simulink model "untitled"  (R2024a)
settings: Solver=VariableStepAuto  StartTime=0.0  StopTime=10.0  RelTol=1e-3
undefined symbols (not defined in the file): x
settings Model: Creator=Hulumulu  LastModifiedBy=Hulumulu

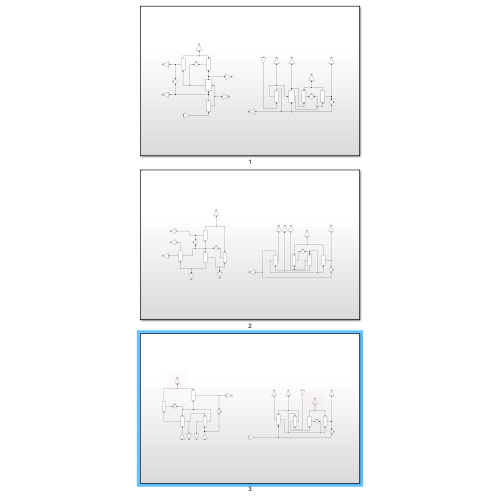
[thumbnail: Simulink's stored preview of the top-level diagram]
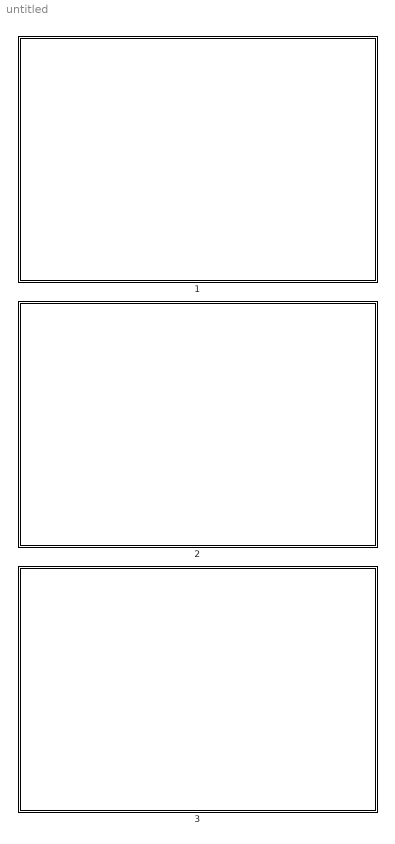
== system untitled ==
  1 : Subsystem
  2 : Subsystem
  3 : Subsystem

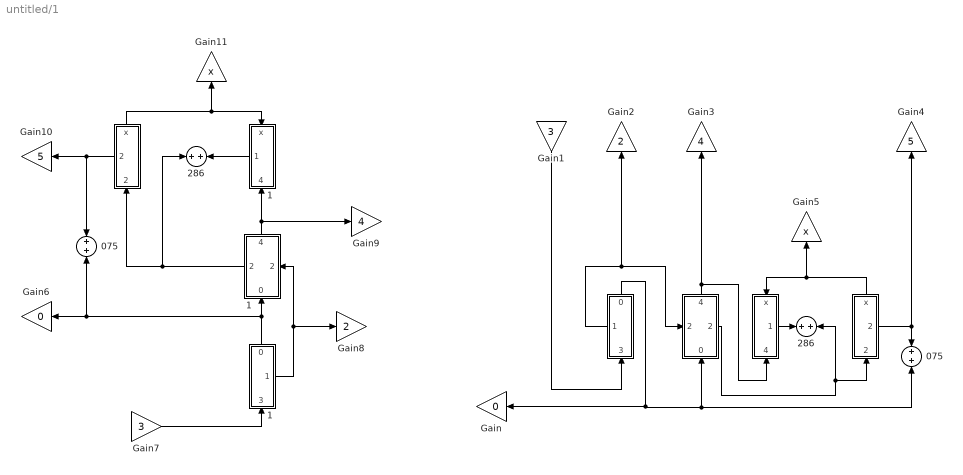
== system untitled/1 ==
  " " : Subsystem
      settings: PortSchema="{\"entries\":[{\"content\":{\"sides\":[{\"content\":{},\"type\":\"ConnectorPlacement.EquallySpacedRectSide\",\"uuid\":\"fb5bb639-39a6-4afc-972d-2ab36dd157e3\"},{\"content\":{\"connectorIds\":[\"Out1\"],\"side\":\"RIGHT\"},\"type\":\"ConnectorPlacement.EquallySpacedRectSide\",\"uuid\":\"d36a19b9-286f-415f-8446-30942908938a\"},{\"content\":{\"connectorIds\":[\"Out2\"],\"side\":\"TOP\"},\"type\":\"ConnectorPlacement.EquallySpacedRectSide\",\"uuid\":\"8c87528f-8b9e-42ba-b050-7318306b7d2b\"},{\"content\":{\"connectorIds\":[\"In1\"],\"side\":\"BOTTOM\"},\"type\":\"ConnectorPlacement.EquallySpacedRectSide\",\"uuid\":\"c4959390-5d76-48db-85f4-dc53d81287e7\"}]},\"type\":\"ConnectorPlacement.EquallySpacedConnector\",\"uuid\":\"3c6f580a-50c2-42c3-8feb-567ef8b292c6\"}],\"packageUris\":[\"http://schema.mathworks.com/mf0/Connector/R2020b\"],\"version\":\"1.0\"}"
  "  " : Subsystem
      settings: PortSchema="{\"entries\":[{\"content\":{\"sides\":[{\"content\":{\"connectorIds\":[\"Out2\"]},\"type\":\"ConnectorPlacement.EquallySpacedRectSide\",\"uuid\":\"fb5bb639-39a6-4afc-972d-2ab36dd157e3\"},{\"content\":{\"connectorIds\":[\"In2\"],\"side\":\"RIGHT\"},\"type\":\"ConnectorPlacement.EquallySpacedRectSide\",\"uuid\":\"d36a19b9-286f-415f-8446-30942908938a\"},{\"content\":{\"connectorIds\":[\"Out1\"],\"side\":\"TOP\"},\"type\":\"ConnectorPlacement.EquallySpacedRectSide\",\"uuid\":\"8c87528f-8b9e-42ba-b050-7318306b7d2b\"},{\"content\":{\"connectorIds\":[\"In1\"],\"side\":\"BOTTOM\"},\"type\":\"ConnectorPlacement.EquallySpacedRectSide\",\"uuid\":\"c4959390-5d76-48db-85f4-dc53d81287e7\"}]},\"type\":\"ConnectorPlacement.EquallySpacedConnector\",\"uuid\":\"3c6f580a-50c2-42c3-8feb-567ef8b292c6\"}],\"packageUris\":[\"http://schema.mathworks.com/mf0/Connector/R2020b\"],\"version\":\"1.0\"}"
  "   " : Subsystem
      settings: PortSchema="{\"entries\":[{\"content\":{\"sides\":[{\"content\":{\"connectorIds\":[\"Out1\"]},\"type\":\"ConnectorPlacement.EquallySpacedRectSide\",\"uuid\":\"fb5bb639-39a6-4afc-972d-2ab36dd157e3\"},{\"content\":{\"side\":\"RIGHT\"},\"type\":\"ConnectorPlacement.EquallySpacedRectSide\",\"uuid\":\"d36a19b9-286f-415f-8446-30942908938a\"},{\"content\":{\"connectorIds\":[\"In1\"],\"side\":\"TOP\"},\"type\":\"ConnectorPlacement.EquallySpacedRectSide\",\"uuid\":\"8c87528f-8b9e-42ba-b050-7318306b7d2b\"},{\"content\":{\"connectorIds\":[\"In2\"],\"side\":\"BOTTOM\"},\"type\":\"ConnectorPlacement.EquallySpacedRectSide\",\"uuid\":\"c4959390-5d76-48db-85f4-dc53d81287e7\"}]},\"type\":\"ConnectorPlacement.EquallySpacedConnector\",\"uuid\":\"3c6f580a-50c2-42c3-8feb-567ef8b292c6\"}],\"packageUris\":[\"http://schema.mathworks.com/mf0/Connector/R2020b\"],\"version\":\"1.0\"}"
  "    " : Subsystem
      settings: PortSchema="{\"entries\":[{\"content\":{\"sides\":[{\"content\":{\"connectorIds\":[\"Out2\"]},\"type\":\"ConnectorPlacement.EquallySpacedRectSide\",\"uuid\":\"fb5bb639-39a6-4afc-972d-2ab36dd157e3\"},{\"content\":{\"side\":\"RIGHT\"},\"type\":\"ConnectorPlacement.EquallySpacedRectSide\",\"uuid\":\"d36a19b9-286f-415f-8446-30942908938a\"},{\"content\":{\"connectorIds\":[\"Out1\"],\"side\":\"TOP\"},\"type\":\"ConnectorPlacement.EquallySpacedRectSide\",\"uuid\":\"8c87528f-8b9e-42ba-b050-7318306b7d2b\"},{\"content\":{\"connectorIds\":[\"In1\"],\"side\":\"BOTTOM\"},\"type\":\"ConnectorPlacement.EquallySpacedRectSide\",\"uuid\":\"c4959390-5d76-48db-85f4-dc53d81287e7\"}]},\"type\":\"ConnectorPlacement.EquallySpacedConnector\",\"uuid\":\"3c6f580a-50c2-42c3-8feb-567ef8b292c6\"}],\"packageUris\":[\"http://schema.mathworks.com/mf0/Connector/R2020b\"],\"version\":\"1.0\"}"
  "     " : Subsystem
      settings: PortSchema="{\"entries\":[{\"content\":{\"sides\":[{\"content\":{\"connectorIds\":[\"Out2\"]},\"type\":\"ConnectorPlacement.EquallySpacedRectSide\",\"uuid\":\"fb5bb639-39a6-4afc-972d-2ab36dd157e3\"},{\"content\":{\"side\":\"RIGHT\"},\"type\":\"ConnectorPlacement.EquallySpacedRectSide\",\"uuid\":\"d36a19b9-286f-415f-8446-30942908938a\"},{\"content\":{\"connectorIds\":[\"Out1\"],\"side\":\"TOP\"},\"type\":\"ConnectorPlacement.EquallySpacedRectSide\",\"uuid\":\"8c87528f-8b9e-42ba-b050-7318306b7d2b\"},{\"content\":{\"connectorIds\":[\"In1\"],\"side\":\"BOTTOM\"},\"type\":\"ConnectorPlacement.EquallySpacedRectSide\",\"uuid\":\"c4959390-5d76-48db-85f4-dc53d81287e7\"}]},\"type\":\"ConnectorPlacement.EquallySpacedConnector\",\"uuid\":\"3c6f580a-50c2-42c3-8feb-567ef8b292c6\"}],\"packageUris\":[\"http://schema.mathworks.com/mf0/Connector/R2020b\"],\"version\":\"1.0\"}"
  "   1" : Subsystem
      settings: PortSchema="{\"entries\":[{\"content\":{\"sides\":[{\"content\":{\"connectorIds\":[\"Out1\"]},\"type\":\"ConnectorPlacement.EquallySpacedRectSide\",\"uuid\":\"fb5bb639-39a6-4afc-972d-2ab36dd157e3\"},{\"content\":{\"side\":\"RIGHT\"},\"type\":\"ConnectorPlacement.EquallySpacedRectSide\",\"uuid\":\"d36a19b9-286f-415f-8446-30942908938a\"},{\"content\":{\"connectorIds\":[\"In1\"],\"side\":\"TOP\"},\"type\":\"ConnectorPlacement.EquallySpacedRectSide\",\"uuid\":\"8c87528f-8b9e-42ba-b050-7318306b7d2b\"},{\"content\":{\"connectorIds\":[\"In2\"],\"side\":\"BOTTOM\"},\"type\":\"ConnectorPlacement.EquallySpacedRectSide\",\"uuid\":\"c4959390-5d76-48db-85f4-dc53d81287e7\"}]},\"type\":\"ConnectorPlacement.EquallySpacedConnector\",\"uuid\":\"3c6f580a-50c2-42c3-8feb-567ef8b292c6\"}],\"packageUris\":[\"http://schema.mathworks.com/mf0/Connector/R2020b\"],\"version\":\"1.0\"}"
  "  1" : Subsystem
      settings: PortSchema="{\"entries\":[{\"content\":{\"sides\":[{\"content\":{\"connectorIds\":[\"Out2\"]},\"type\":\"ConnectorPlacement.EquallySpacedRectSide\",\"uuid\":\"fb5bb639-39a6-4afc-972d-2ab36dd157e3\"},{\"content\":{\"connectorIds\":[\"In2\"],\"side\":\"RIGHT\"},\"type\":\"ConnectorPlacement.EquallySpacedRectSide\",\"uuid\":\"d36a19b9-286f-415f-8446-30942908938a\"},{\"content\":{\"connectorIds\":[\"Out1\"],\"side\":\"TOP\"},\"type\":\"ConnectorPlacement.EquallySpacedRectSide\",\"uuid\":\"8c87528f-8b9e-42ba-b050-7318306b7d2b\"},{\"content\":{\"connectorIds\":[\"In1\"],\"side\":\"BOTTOM\"},\"type\":\"ConnectorPlacement.EquallySpacedRectSide\",\"uuid\":\"c4959390-5d76-48db-85f4-dc53d81287e7\"}]},\"type\":\"ConnectorPlacement.EquallySpacedConnector\",\"uuid\":\"3c6f580a-50c2-42c3-8feb-567ef8b292c6\"}],\"packageUris\":[\"http://schema.mathworks.com/mf0/Connector/R2020b\"],\"version\":\"1.0\"}"
  " 1" : Subsystem
      settings: PortSchema="{\"entries\":[{\"content\":{\"sides\":[{\"content\":{},\"type\":\"ConnectorPlacement.EquallySpacedRectSide\",\"uuid\":\"fb5bb639-39a6-4afc-972d-2ab36dd157e3\"},{\"content\":{\"connectorIds\":[\"Out1\"],\"side\":\"RIGHT\"},\"type\":\"ConnectorPlacement.EquallySpacedRectSide\",\"uuid\":\"d36a19b9-286f-415f-8446-30942908938a\"},{\"content\":{\"connectorIds\":[\"Out2\"],\"side\":\"TOP\"},\"type\":\"ConnectorPlacement.EquallySpacedRectSide\",\"uuid\":\"8c87528f-8b9e-42ba-b050-7318306b7d2b\"},{\"content\":{\"connectorIds\":[\"In1\"],\"side\":\"BOTTOM\"},\"type\":\"ConnectorPlacement.EquallySpacedRectSide\",\"uuid\":\"c4959390-5d76-48db-85f4-dc53d81287e7\"}]},\"type\":\"ConnectorPlacement.EquallySpacedConnector\",\"uuid\":\"3c6f580a-50c2-42c3-8feb-567ef8b292c6\"}],\"packageUris\":[\"http://schema.mathworks.com/mf0/Connector/R2020b\"],\"version\":\"1.0\"}"
  075 : Sum  Inputs=+|+
  "075 " : Sum  Inputs=+|+
  286 : Sum  Inputs=+|+
  "286 " : Sum  Inputs=+|+
  Gain : Gain  Gain=0
  Gain1 : Gain  Gain=3
  Gain10 : Gain  Gain=5
  Gain11 : Gain  Gain=x
  Gain2 : Gain  Gain=2
  Gain3 : Gain  Gain=4
  Gain4 : Gain  Gain=5
  Gain5 : Gain  Gain=x
  Gain6 : Gain  Gain=0
  Gain7 : Gain  Gain=3
  Gain8 : Gain  Gain=2
  Gain9 : Gain  Gain=4
  wires:
  " "/1(2) -> "  "/2("2 "), Gain2/1
  "  "/2(2) -> "    "/1(2), 286/2
  "  "/1(4) -> "   "/2(4), Gain3/1
  "    "/1(x) -> Gain5/1, "   "/1(x)
  Gain1/1 -> " "/1(3)
  "   "/1(6) -> 286/1
  "    "/2(5) -> Gain4/1, 075/1
  " "/2(0) -> "  "/1(0), 075/2, Gain/1
  Gain7/1 -> " 1"/1(3)
  "     "/2(5) -> "075 "/1, Gain10/1
  "   1"/1(6) -> "286 "/2
  "  1"/1(4) -> Gain9/1, "   1"/2(4)
  "     "/1(x) -> Gain11/1, "   1"/1(x)
  " 1"/1(2) -> "  1"/2("2 "), Gain8/1
  " 1"/2(0) -> "075 "/2, Gain6/1, "  1"/1(0)
  "  1"/2(2) -> "286 "/1, "     "/1(2)

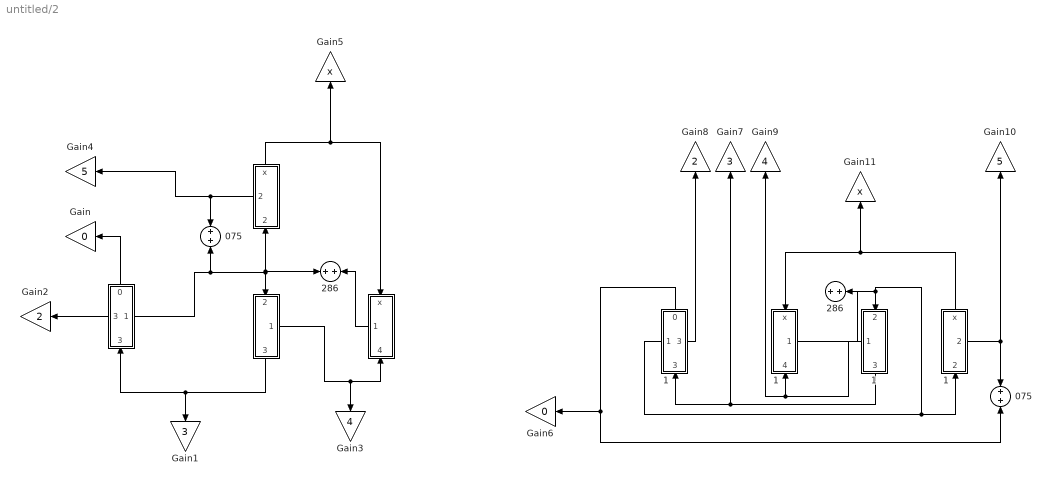
== system untitled/2 ==
  " " : Subsystem
      settings: PortSchema="{\"entries\":[{\"content\":{\"sides\":[{\"content\":{\"connectorIds\":[\"Out3\"]},\"type\":\"ConnectorPlacement.EquallySpacedRectSide\",\"uuid\":\"fb5bb639-39a6-4afc-972d-2ab36dd157e3\"},{\"content\":{\"connectorIds\":[\"Out1\"],\"side\":\"RIGHT\"},\"type\":\"ConnectorPlacement.EquallySpacedRectSide\",\"uuid\":\"d36a19b9-286f-415f-8446-30942908938a\"},{\"content\":{\"connectorIds\":[\"Out2\"],\"side\":\"TOP\"},\"type\":\"ConnectorPlacement.EquallySpacedRectSide\",\"uuid\":\"8c87528f-8b9e-42ba-b050-7318306b7d2b\"},{\"content\":{\"connectorIds\":[\"In1\"],\"side\":\"BOTTOM\"},\"type\":\"ConnectorPlacement.EquallySpacedRectSide\",\"uuid\":\"c4959390-5d76-48db-85f4-dc53d81287e7\"}]},\"type\":\"ConnectorPlacement.EquallySpacedConnector\",\"uuid\":\"3c6f580a-50c2-42c3-8feb-567ef8b292c6\"}],\"packageUris\":[\"http://schema.mathworks.com/mf0/Connector/R2020b\"],\"version\":\"1.0\"}"
  "   " : Subsystem
      settings: PortSchema="{\"entries\":[{\"content\":{\"sides\":[{\"content\":{\"connectorIds\":[\"Out1\"]},\"type\":\"ConnectorPlacement.EquallySpacedRectSide\",\"uuid\":\"fb5bb639-39a6-4afc-972d-2ab36dd157e3\"},{\"content\":{\"side\":\"RIGHT\"},\"type\":\"ConnectorPlacement.EquallySpacedRectSide\",\"uuid\":\"d36a19b9-286f-415f-8446-30942908938a\"},{\"content\":{\"connectorIds\":[\"In1\"],\"side\":\"TOP\"},\"type\":\"ConnectorPlacement.EquallySpacedRectSide\",\"uuid\":\"8c87528f-8b9e-42ba-b050-7318306b7d2b\"},{\"content\":{\"connectorIds\":[\"In2\"],\"side\":\"BOTTOM\"},\"type\":\"ConnectorPlacement.EquallySpacedRectSide\",\"uuid\":\"c4959390-5d76-48db-85f4-dc53d81287e7\"}]},\"type\":\"ConnectorPlacement.EquallySpacedConnector\",\"uuid\":\"3c6f580a-50c2-42c3-8feb-567ef8b292c6\"}],\"packageUris\":[\"http://schema.mathworks.com/mf0/Connector/R2020b\"],\"version\":\"1.0\"}"
  "    " : Subsystem
      settings: PortSchema="{\"entries\":[{\"content\":{\"sides\":[{\"content\":{\"connectorIds\":[\"Out2\"]},\"type\":\"ConnectorPlacement.EquallySpacedRectSide\",\"uuid\":\"fb5bb639-39a6-4afc-972d-2ab36dd157e3\"},{\"content\":{\"side\":\"RIGHT\"},\"type\":\"ConnectorPlacement.EquallySpacedRectSide\",\"uuid\":\"d36a19b9-286f-415f-8446-30942908938a\"},{\"content\":{\"connectorIds\":[\"Out1\"],\"side\":\"TOP\"},\"type\":\"ConnectorPlacement.EquallySpacedRectSide\",\"uuid\":\"8c87528f-8b9e-42ba-b050-7318306b7d2b\"},{\"content\":{\"connectorIds\":[\"In1\"],\"side\":\"BOTTOM\"},\"type\":\"ConnectorPlacement.EquallySpacedRectSide\",\"uuid\":\"c4959390-5d76-48db-85f4-dc53d81287e7\"}]},\"type\":\"ConnectorPlacement.EquallySpacedConnector\",\"uuid\":\"3c6f580a-50c2-42c3-8feb-567ef8b292c6\"}],\"packageUris\":[\"http://schema.mathworks.com/mf0/Connector/R2020b\"],\"version\":\"1.0\"}"
  "     " : Subsystem
      settings: PortSchema="{\"entries\":[{\"content\":{\"sides\":[{\"content\":{},\"type\":\"ConnectorPlacement.EquallySpacedRectSide\",\"uuid\":\"fb5bb639-39a6-4afc-972d-2ab36dd157e3\"},{\"content\":{\"connectorIds\":[\"Out1\"],\"side\":\"RIGHT\"},\"type\":\"ConnectorPlacement.EquallySpacedRectSide\",\"uuid\":\"d36a19b9-286f-415f-8446-30942908938a\"},{\"content\":{\"connectorIds\":[\"In1\"],\"side\":\"TOP\"},\"type\":\"ConnectorPlacement.EquallySpacedRectSide\",\"uuid\":\"8c87528f-8b9e-42ba-b050-7318306b7d2b\"},{\"content\":{\"connectorIds\":[\"Out2\"],\"side\":\"BOTTOM\"},\"type\":\"ConnectorPlacement.EquallySpacedRectSide\",\"uuid\":\"c4959390-5d76-48db-85f4-dc53d81287e7\"}]},\"type\":\"ConnectorPlacement.EquallySpacedConnector\",\"uuid\":\"3c6f580a-50c2-42c3-8feb-567ef8b292c6\"}],\"packageUris\":[\"http://schema.mathworks.com/mf0/Connector/R2020b\"],\"version\":\"1.0\"}"
  "     1" : Subsystem
      settings: PortSchema="{\"entries\":[{\"content\":{\"sides\":[{\"content\":{},\"type\":\"ConnectorPlacement.EquallySpacedRectSide\",\"uuid\":\"fb5bb639-39a6-4afc-972d-2ab36dd157e3\"},{\"content\":{\"connectorIds\":[\"Out1\"],\"side\":\"RIGHT\"},\"type\":\"ConnectorPlacement.EquallySpacedRectSide\",\"uuid\":\"d36a19b9-286f-415f-8446-30942908938a\"},{\"content\":{\"connectorIds\":[\"In1\"],\"side\":\"TOP\"},\"type\":\"ConnectorPlacement.EquallySpacedRectSide\",\"uuid\":\"8c87528f-8b9e-42ba-b050-7318306b7d2b\"},{\"content\":{\"connectorIds\":[\"Out2\"],\"side\":\"BOTTOM\"},\"type\":\"ConnectorPlacement.EquallySpacedRectSide\",\"uuid\":\"c4959390-5d76-48db-85f4-dc53d81287e7\"}]},\"type\":\"ConnectorPlacement.EquallySpacedConnector\",\"uuid\":\"3c6f580a-50c2-42c3-8feb-567ef8b292c6\"}],\"packageUris\":[\"http://schema.mathworks.com/mf0/Connector/R2020b\"],\"version\":\"1.0\"}"
  "    1" : Subsystem
      settings: PortSchema="{\"entries\":[{\"content\":{\"sides\":[{\"content\":{\"connectorIds\":[\"Out2\"]},\"type\":\"ConnectorPlacement.EquallySpacedRectSide\",\"uuid\":\"fb5bb639-39a6-4afc-972d-2ab36dd157e3\"},{\"content\":{\"side\":\"RIGHT\"},\"type\":\"ConnectorPlacement.EquallySpacedRectSide\",\"uuid\":\"d36a19b9-286f-415f-8446-30942908938a\"},{\"content\":{\"connectorIds\":[\"Out1\"],\"side\":\"TOP\"},\"type\":\"ConnectorPlacement.EquallySpacedRectSide\",\"uuid\":\"8c87528f-8b9e-42ba-b050-7318306b7d2b\"},{\"content\":{\"connectorIds\":[\"In1\"],\"side\":\"BOTTOM\"},\"type\":\"ConnectorPlacement.EquallySpacedRectSide\",\"uuid\":\"c4959390-5d76-48db-85f4-dc53d81287e7\"}]},\"type\":\"ConnectorPlacement.EquallySpacedConnector\",\"uuid\":\"3c6f580a-50c2-42c3-8feb-567ef8b292c6\"}],\"packageUris\":[\"http://schema.mathworks.com/mf0/Connector/R2020b\"],\"version\":\"1.0\"}"
  "   1" : Subsystem
      settings: PortSchema="{\"entries\":[{\"content\":{\"sides\":[{\"content\":{\"connectorIds\":[\"Out1\"]},\"type\":\"ConnectorPlacement.EquallySpacedRectSide\",\"uuid\":\"fb5bb639-39a6-4afc-972d-2ab36dd157e3\"},{\"content\":{\"side\":\"RIGHT\"},\"type\":\"ConnectorPlacement.EquallySpacedRectSide\",\"uuid\":\"d36a19b9-286f-415f-8446-30942908938a\"},{\"content\":{\"connectorIds\":[\"In1\"],\"side\":\"TOP\"},\"type\":\"ConnectorPlacement.EquallySpacedRectSide\",\"uuid\":\"8c87528f-8b9e-42ba-b050-7318306b7d2b\"},{\"content\":{\"connectorIds\":[\"In2\"],\"side\":\"BOTTOM\"},\"type\":\"ConnectorPlacement.EquallySpacedRectSide\",\"uuid\":\"c4959390-5d76-48db-85f4-dc53d81287e7\"}]},\"type\":\"ConnectorPlacement.EquallySpacedConnector\",\"uuid\":\"3c6f580a-50c2-42c3-8feb-567ef8b292c6\"}],\"packageUris\":[\"http://schema.mathworks.com/mf0/Connector/R2020b\"],\"version\":\"1.0\"}"
  " 1" : Subsystem
      settings: PortSchema="{\"entries\":[{\"content\":{\"sides\":[{\"content\":{\"connectorIds\":[\"Out3\"]},\"type\":\"ConnectorPlacement.EquallySpacedRectSide\",\"uuid\":\"fb5bb639-39a6-4afc-972d-2ab36dd157e3\"},{\"content\":{\"connectorIds\":[\"Out1\"],\"side\":\"RIGHT\"},\"type\":\"ConnectorPlacement.EquallySpacedRectSide\",\"uuid\":\"d36a19b9-286f-415f-8446-30942908938a\"},{\"content\":{\"connectorIds\":[\"Out2\"],\"side\":\"TOP\"},\"type\":\"ConnectorPlacement.EquallySpacedRectSide\",\"uuid\":\"8c87528f-8b9e-42ba-b050-7318306b7d2b\"},{\"content\":{\"connectorIds\":[\"In1\"],\"side\":\"BOTTOM\"},\"type\":\"ConnectorPlacement.EquallySpacedRectSide\",\"uuid\":\"c4959390-5d76-48db-85f4-dc53d81287e7\"}]},\"type\":\"ConnectorPlacement.EquallySpacedConnector\",\"uuid\":\"3c6f580a-50c2-42c3-8feb-567ef8b292c6\"}],\"packageUris\":[\"http://schema.mathworks.com/mf0/Connector/R2020b\"],\"version\":\"1.0\"}"
  075 : Sum  Inputs=+|+
  "075  " : Sum  Inputs=+|+
  286 : Sum  Inputs=+|+
  "286  " : Sum  Inputs=+|+
  Gain : Gain  Gain=0
  Gain1 : Gain  Gain=3
  Gain10 : Gain  Gain=5
  Gain11 : Gain  Gain=x
  Gain2 : Gain  Gain=2
  Gain3 : Gain  Gain=4
  Gain4 : Gain  Gain=5
  Gain5 : Gain  Gain=x
  Gain6 : Gain  Gain=0
  Gain7 : Gain  Gain=3
  Gain8 : Gain  Gain=2
  Gain9 : Gain  Gain=4
  wires:
  " "/2(0) -> Gain/1
  " "/3("2 ") -> Gain2/1
  "     "/2(3) -> Gain1/1, " "/1(3)
  "     "/1(4) -> "   "/2(4), Gain3/1
  " "/1(2) -> "    "/1(2), 286/1, "     "/1(2), 075/2
  "    "/1(x) -> "   "/1(x), Gain5/1
  "    "/2(5) -> Gain4/1, 075/1
  "   "/1(6) -> 286/2
  "    1"/1(x) -> Gain11/1, "   1"/1(x)
  " 1"/1(2) -> "    1"/1(2), "     1"/1(2), "286  "/2
  "    1"/2(5) -> "075  "/1, Gain10/1
  " 1"/2(0) -> "075  "/2, Gain6/1
  " 1"/3("2 ") -> Gain8/1
  "     1"/2(3) -> " 1"/1(3), Gain7/1
  "     1"/1(4) -> "   1"/2(4), Gain9/1
  "   1"/1(6) -> "286  "/1

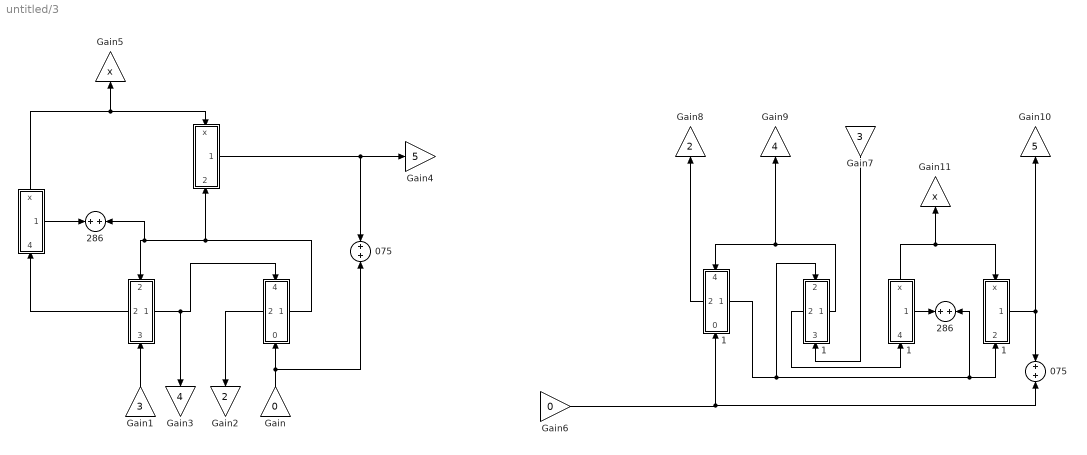
== system untitled/3 ==
  "  " : Subsystem
      settings: PortSchema="{\"entries\":[{\"content\":{\"sides\":[{\"content\":{\"connectorIds\":[\"Out2\"]},\"type\":\"ConnectorPlacement.EquallySpacedRectSide\",\"uuid\":\"fb5bb639-39a6-4afc-972d-2ab36dd157e3\"},{\"content\":{\"connectorIds\":[\"Out1\"],\"side\":\"RIGHT\"},\"type\":\"ConnectorPlacement.EquallySpacedRectSide\",\"uuid\":\"d36a19b9-286f-415f-8446-30942908938a\"},{\"content\":{\"connectorIds\":[\"In1\"],\"side\":\"TOP\"},\"type\":\"ConnectorPlacement.EquallySpacedRectSide\",\"uuid\":\"8c87528f-8b9e-42ba-b050-7318306b7d2b\"},{\"content\":{\"connectorIds\":[\"In2\"],\"side\":\"BOTTOM\"},\"type\":\"ConnectorPlacement.EquallySpacedRectSide\",\"uuid\":\"c4959390-5d76-48db-85f4-dc53d81287e7\"}]},\"type\":\"ConnectorPlacement.EquallySpacedConnector\",\"uuid\":\"3c6f580a-50c2-42c3-8feb-567ef8b292c6\"}],\"packageUris\":[\"http://schema.mathworks.com/mf0/Connector/R2020b\"],\"version\":\"1.0\"}"
  "   " : Subsystem
      settings: PortSchema="{\"entries\":[{\"content\":{\"sides\":[{\"content\":{},\"type\":\"ConnectorPlacement.EquallySpacedRectSide\",\"uuid\":\"fb5bb639-39a6-4afc-972d-2ab36dd157e3\"},{\"content\":{\"connectorIds\":[\"Out1\"],\"side\":\"RIGHT\"},\"type\":\"ConnectorPlacement.EquallySpacedRectSide\",\"uuid\":\"d36a19b9-286f-415f-8446-30942908938a\"},{\"content\":{\"connectorIds\":[\"Out2\"],\"side\":\"TOP\"},\"type\":\"ConnectorPlacement.EquallySpacedRectSide\",\"uuid\":\"8c87528f-8b9e-42ba-b050-7318306b7d2b\"},{\"content\":{\"connectorIds\":[\"In1\"],\"side\":\"BOTTOM\"},\"type\":\"ConnectorPlacement.EquallySpacedRectSide\",\"uuid\":\"c4959390-5d76-48db-85f4-dc53d81287e7\"}]},\"type\":\"ConnectorPlacement.EquallySpacedConnector\",\"uuid\":\"3c6f580a-50c2-42c3-8feb-567ef8b292c6\"}],\"packageUris\":[\"http://schema.mathworks.com/mf0/Connector/R2020b\"],\"version\":\"1.0\"}"
  "    " : Subsystem
      settings: PortSchema="{\"entries\":[{\"content\":{\"sides\":[{\"content\":{},\"type\":\"ConnectorPlacement.EquallySpacedRectSide\",\"uuid\":\"fb5bb639-39a6-4afc-972d-2ab36dd157e3\"},{\"content\":{\"connectorIds\":[\"Out1\"],\"side\":\"RIGHT\"},\"type\":\"ConnectorPlacement.EquallySpacedRectSide\",\"uuid\":\"d36a19b9-286f-415f-8446-30942908938a\"},{\"content\":{\"connectorIds\":[\"In1\"],\"side\":\"TOP\"},\"type\":\"ConnectorPlacement.EquallySpacedRectSide\",\"uuid\":\"8c87528f-8b9e-42ba-b050-7318306b7d2b\"},{\"content\":{\"connectorIds\":[\"In2\"],\"side\":\"BOTTOM\"},\"type\":\"ConnectorPlacement.EquallySpacedRectSide\",\"uuid\":\"c4959390-5d76-48db-85f4-dc53d81287e7\"}]},\"type\":\"ConnectorPlacement.EquallySpacedConnector\",\"uuid\":\"3c6f580a-50c2-42c3-8feb-567ef8b292c6\"}],\"packageUris\":[\"http://schema.mathworks.com/mf0/Connector/R2020b\"],\"version\":\"1.0\"}"
  "     " : Subsystem
      settings: PortSchema="{\"entries\":[{\"content\":{\"sides\":[{\"content\":{\"connectorIds\":[\"Out2\"]},\"type\":\"ConnectorPlacement.EquallySpacedRectSide\",\"uuid\":\"fb5bb639-39a6-4afc-972d-2ab36dd157e3\"},{\"content\":{\"connectorIds\":[\"Out1\"],\"side\":\"RIGHT\"},\"type\":\"ConnectorPlacement.EquallySpacedRectSide\",\"uuid\":\"d36a19b9-286f-415f-8446-30942908938a\"},{\"content\":{\"connectorIds\":[\"In1\"],\"side\":\"TOP\"},\"type\":\"ConnectorPlacement.EquallySpacedRectSide\",\"uuid\":\"8c87528f-8b9e-42ba-b050-7318306b7d2b\"},{\"content\":{\"connectorIds\":[\"In2\"],\"side\":\"BOTTOM\"},\"type\":\"ConnectorPlacement.EquallySpacedRectSide\",\"uuid\":\"c4959390-5d76-48db-85f4-dc53d81287e7\"}]},\"type\":\"ConnectorPlacement.EquallySpacedConnector\",\"uuid\":\"3c6f580a-50c2-42c3-8feb-567ef8b292c6\"}],\"packageUris\":[\"http://schema.mathworks.com/mf0/Connector/R2020b\"],\"version\":\"1.0\"}"
  "     1" : Subsystem
      settings: PortSchema="{\"entries\":[{\"content\":{\"sides\":[{\"content\":{\"connectorIds\":[\"Out2\"]},\"type\":\"ConnectorPlacement.EquallySpacedRectSide\",\"uuid\":\"fb5bb639-39a6-4afc-972d-2ab36dd157e3\"},{\"content\":{\"connectorIds\":[\"Out1\"],\"side\":\"RIGHT\"},\"type\":\"ConnectorPlacement.EquallySpacedRectSide\",\"uuid\":\"d36a19b9-286f-415f-8446-30942908938a\"},{\"content\":{\"connectorIds\":[\"In1\"],\"side\":\"TOP\"},\"type\":\"ConnectorPlacement.EquallySpacedRectSide\",\"uuid\":\"8c87528f-8b9e-42ba-b050-7318306b7d2b\"},{\"content\":{\"connectorIds\":[\"In2\"],\"side\":\"BOTTOM\"},\"type\":\"ConnectorPlacement.EquallySpacedRectSide\",\"uuid\":\"c4959390-5d76-48db-85f4-dc53d81287e7\"}]},\"type\":\"ConnectorPlacement.EquallySpacedConnector\",\"uuid\":\"3c6f580a-50c2-42c3-8feb-567ef8b292c6\"}],\"packageUris\":[\"http://schema.mathworks.com/mf0/Connector/R2020b\"],\"version\":\"1.0\"}"
  "    1" : Subsystem
      settings: PortSchema="{\"entries\":[{\"content\":{\"sides\":[{\"content\":{},\"type\":\"ConnectorPlacement.EquallySpacedRectSide\",\"uuid\":\"fb5bb639-39a6-4afc-972d-2ab36dd157e3\"},{\"content\":{\"connectorIds\":[\"Out1\"],\"side\":\"RIGHT\"},\"type\":\"ConnectorPlacement.EquallySpacedRectSide\",\"uuid\":\"d36a19b9-286f-415f-8446-30942908938a\"},{\"content\":{\"connectorIds\":[\"In1\"],\"side\":\"TOP\"},\"type\":\"ConnectorPlacement.EquallySpacedRectSide\",\"uuid\":\"8c87528f-8b9e-42ba-b050-7318306b7d2b\"},{\"content\":{\"connectorIds\":[\"In2\"],\"side\":\"BOTTOM\"},\"type\":\"ConnectorPlacement.EquallySpacedRectSide\",\"uuid\":\"c4959390-5d76-48db-85f4-dc53d81287e7\"}]},\"type\":\"ConnectorPlacement.EquallySpacedConnector\",\"uuid\":\"3c6f580a-50c2-42c3-8feb-567ef8b292c6\"}],\"packageUris\":[\"http://schema.mathworks.com/mf0/Connector/R2020b\"],\"version\":\"1.0\"}"
  "   1" : Subsystem
      settings: PortSchema="{\"entries\":[{\"content\":{\"sides\":[{\"content\":{},\"type\":\"ConnectorPlacement.EquallySpacedRectSide\",\"uuid\":\"fb5bb639-39a6-4afc-972d-2ab36dd157e3\"},{\"content\":{\"connectorIds\":[\"Out1\"],\"side\":\"RIGHT\"},\"type\":\"ConnectorPlacement.EquallySpacedRectSide\",\"uuid\":\"d36a19b9-286f-415f-8446-30942908938a\"},{\"content\":{\"connectorIds\":[\"Out2\"],\"side\":\"TOP\"},\"type\":\"ConnectorPlacement.EquallySpacedRectSide\",\"uuid\":\"8c87528f-8b9e-42ba-b050-7318306b7d2b\"},{\"content\":{\"connectorIds\":[\"In1\"],\"side\":\"BOTTOM\"},\"type\":\"ConnectorPlacement.EquallySpacedRectSide\",\"uuid\":\"c4959390-5d76-48db-85f4-dc53d81287e7\"}]},\"type\":\"ConnectorPlacement.EquallySpacedConnector\",\"uuid\":\"3c6f580a-50c2-42c3-8feb-567ef8b292c6\"}],\"packageUris\":[\"http://schema.mathworks.com/mf0/Connector/R2020b\"],\"version\":\"1.0\"}"
  "  1" : Subsystem
      settings: PortSchema="{\"entries\":[{\"content\":{\"sides\":[{\"content\":{\"connectorIds\":[\"Out2\"]},\"type\":\"ConnectorPlacement.EquallySpacedRectSide\",\"uuid\":\"fb5bb639-39a6-4afc-972d-2ab36dd157e3\"},{\"content\":{\"connectorIds\":[\"Out1\"],\"side\":\"RIGHT\"},\"type\":\"ConnectorPlacement.EquallySpacedRectSide\",\"uuid\":\"d36a19b9-286f-415f-8446-30942908938a\"},{\"content\":{\"connectorIds\":[\"In1\"],\"side\":\"TOP\"},\"type\":\"ConnectorPlacement.EquallySpacedRectSide\",\"uuid\":\"8c87528f-8b9e-42ba-b050-7318306b7d2b\"},{\"content\":{\"connectorIds\":[\"In2\"],\"side\":\"BOTTOM\"},\"type\":\"ConnectorPlacement.EquallySpacedRectSide\",\"uuid\":\"c4959390-5d76-48db-85f4-dc53d81287e7\"}]},\"type\":\"ConnectorPlacement.EquallySpacedConnector\",\"uuid\":\"3c6f580a-50c2-42c3-8feb-567ef8b292c6\"}],\"packageUris\":[\"http://schema.mathworks.com/mf0/Connector/R2020b\"],\"version\":\"1.0\"}"
  075 : Sum  Inputs=+|+
  "075 " : Sum  Inputs=+|+
  286 : Sum  Inputs=+|+
  "286 " : Sum  Inputs=+|+
  Gain : Gain  Gain=0
  Gain1 : Gain  Gain=3
  Gain10 : Gain  Gain=5
  Gain11 : Gain  Gain=x
  Gain2 : Gain  Gain=2
  Gain3 : Gain  Gain=4
  Gain4 : Gain  Gain=5
  Gain5 : Gain  Gain=x
  Gain6 : Gain  Gain=0
  Gain7 : Gain  Gain=3
  Gain8 : Gain  Gain=2
  Gain9 : Gain  Gain=4
  wires:
  Gain/1 -> 075/2, "  "/2(0)
  "  "/2("2 ") -> Gain2/1
  "  "/1(2) -> 286/2, "     "/1(2), "    "/2(2)
  "   "/1(6) -> 286/1
  "    "/1(5) -> 075/1, Gain4/1
  "     "/1(4) -> Gain3/1, "  "/1(4)
  Gain1/1 -> "     "/2(3)
  "     "/2("4 ") -> "   "/1(4)
  "   "/2(x) -> Gain5/1, "    "/1(x)
  "  1"/2("2 ") -> Gain8/1
  "   1"/2(x) -> "    1"/1(x), Gain11/1
  "     1"/2("4 ") -> "   1"/1(4)
  Gain6/1 -> "  1"/2(0), "075 "/2
  "     1"/1(4) -> Gain9/1, "  1"/1(4)
  "    1"/1(5) -> "075 "/1, Gain10/1
  "  1"/1(2) -> "286 "/2, "    1"/2(2), "     1"/1(2)
  Gain7/1 -> "     1"/2(3)
  "   1"/1(6) -> "286 "/1

== system untitled/1/  ==
  3 : Inport
  2 : Outport
  0 : Outport  Port=2
  wires:
  3/1 -> 2/1, 0/1

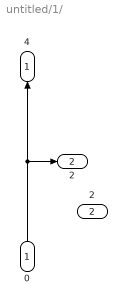
== system untitled/1/   ==
  0 : Inport
  "2 " : Inport  Port=2
  4 : Outport
  2 : Outport  Port=2
  wires:
  0/1 -> 4/1, 2/1

== system untitled/1/    ==
  x : Inport
  4 : Inport  Port=2
  6 : Outport
  wires:
  4/1 -> 6/1

== system untitled/1/     ==
  2 : Inport
  x : Outport
  5 : Outport  Port=2
  wires:
  2/1 -> x/1, 5/1

== system untitled/1/      ==
  2 : Inport
  x : Outport
  5 : Outport  Port=2
  wires:
  2/1 -> x/1, 5/1

== system untitled/1/   1 ==
  x : Inport
  4 : Inport  Port=2
  6 : Outport
  wires:
  4/1 -> 6/1

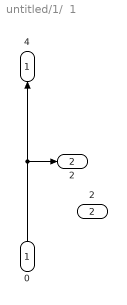
== system untitled/1/  1 ==
  0 : Inport
  "2 " : Inport  Port=2
  4 : Outport
  2 : Outport  Port=2
  wires:
  0/1 -> 4/1, 2/1

== system untitled/1/ 1 ==
  3 : Inport
  2 : Outport
  0 : Outport  Port=2
  wires:
  3/1 -> 2/1, 0/1

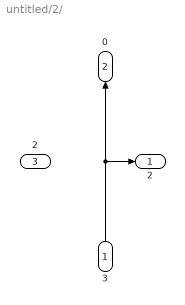
== system untitled/2/  ==
  3 : Inport
  2 : Outport
  0 : Outport  Port=2
  "2 " : Outport  Port=3
  wires:
  3/1 -> 0/1, 2/1

== system untitled/2/    ==
  x : Inport
  4 : Inport  Port=2
  6 : Outport
  wires:
  4/1 -> 6/1

== system untitled/2/     ==
  2 : Inport
  x : Outport
  5 : Outport  Port=2
  wires:
  2/1 -> 5/1, x/1

== system untitled/2/      ==
  2 : Inport
  4 : Outport
  3 : Outport  Port=2

== system untitled/2/     1 ==
  2 : Inport
  4 : Outport
  3 : Outport  Port=2

== system untitled/2/    1 ==
  2 : Inport
  x : Outport
  5 : Outport  Port=2
  wires:
  2/1 -> 5/1, x/1

== system untitled/2/   1 ==
  x : Inport
  4 : Inport  Port=2
  6 : Outport
  wires:
  4/1 -> 6/1

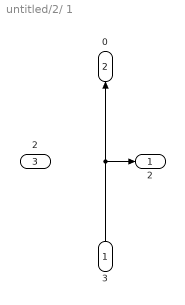
== system untitled/2/ 1 ==
  3 : Inport
  2 : Outport
  0 : Outport  Port=2
  "2 " : Outport  Port=3
  wires:
  3/1 -> 0/1, 2/1

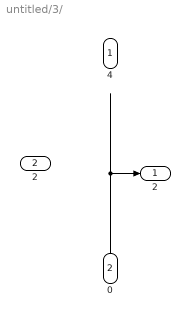
== system untitled/3/   ==
  4 : Inport
  0 : Inport  Port=2
  2 : Outport
  "2 " : Outport  Port=2
  wires:
  0/1 -> 2/1

== system untitled/3/    ==
  4 : Inport
  6 : Outport
  x : Outport  Port=2
  wires:
  4/1 -> 6/1, x/1

== system untitled/3/     ==
  x : Inport
  2 : Inport  Port=2
  5 : Outport
  wires:
  2/1 -> 5/1

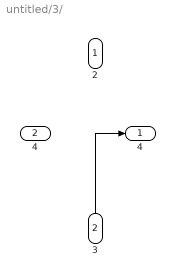
== system untitled/3/      ==
  2 : Inport
  3 : Inport  Port=2
  4 : Outport
  "4 " : Outport  Port=2
  wires:
  3/1 -> 4/1

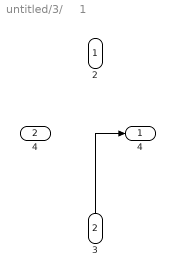
== system untitled/3/     1 ==
  2 : Inport
  3 : Inport  Port=2
  4 : Outport
  "4 " : Outport  Port=2
  wires:
  3/1 -> 4/1

== system untitled/3/    1 ==
  x : Inport
  2 : Inport  Port=2
  5 : Outport
  wires:
  2/1 -> 5/1

== system untitled/3/   1 ==
  4 : Inport
  6 : Outport
  x : Outport  Port=2
  wires:
  4/1 -> 6/1, x/1

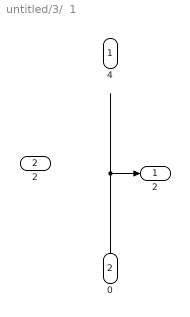
== system untitled/3/  1 ==
  4 : Inport
  0 : Inport  Port=2
  2 : Outport
  "2 " : Outport  Port=2
  wires:
  0/1 -> 2/1
